simulink model "HD2_Driver_PY_v3"  (R2018a)
settings: Solver=ode1  StartTime=0.0  StopTime=inf  FixedStep=0.001  RelTol=1e-3  EnableMultiTasking=on
InitFcn:
  | % Assign block mask parameter to variable in base workspace
  | mdlPrefix_hd2_py = 'HD2_PY_';
  | mdlName_hd2_py = 'HD2_Driver_PY_v3';
  | blkName_hd2_py = 'HD2_Parameters';
  | blkRef_hd2_py = strcat(mdlName_hd2_py, '/', blkName_hd2_py);
  | 
  | % Extract list of parameters defined in the "HD2 Parameter" subsystem block
  | dialogParams_hd2_py = get_param( blkRef_hd2_py,'DialogParameters');
  | dialogParamsNames_hd2_py = fieldnames(dialogParams_hd2_py);
  | 
  | % Assign each parameter to a variable with mdlPrefix<param_name> formatted name
  | for idx = 1:numel(dialogParamsNames_hd2_py)
  |     paramVal = eval( get_param( blkRef_hd2_py, dialogParamsNames_hd2_py{idx} ) );
  |     assignin( 'base', strcat(mdlPrefix_hd2_py,dialogParamsNames_hd2_py{idx}), paramVal);
  | end
  | 
model workspace (MAT data in the model file):
  MCOS : class17 (value not decoded)
undefined symbols (not defined in the file): HD2_PY_CalibHome, HD2_PY_HandleLength, HD2_PY_HandleOffset, HD2_PY_HandleTol, HD2_PY_LinkLengths, HD2_PY_MotorAmpGains, HD2_PY_MotorAmpLimits, HD2_PY_QDirs, HD2_PY_QEnc, HD2_PY_QGains, HD2_PY_QKv, HIL, qc_get_step_size
libraries: quarc_library x30, simulink x10, simulink_extras x6
(part 2 of 2)

== matlab function HD2_Driver_PY_v3/Five Bar (PY) - Upper ==
  data: q input; Pos output; LinkLengths input; J output; R output
function [Pos, J, R] = FiveBarKinematics_PY(q, LinkLengths)
%#codegen

% This function computes the kinematics for a 5-Bar Mechanism (POSITIVE Y).

% The 5-Bar has three joints:
% Base Joint (q1): Defined to be rotating about the 5-Bar Native/Inertial x-axis
% First Joint (q2): Defined to be rotating about the local z-axis (when q1=0)
% Second Joint (q3): Also rotating about the local z-axis (when q1=0)
%
% The frames are defined such that when q=[0,0,0], the upper links are
% extending out towards the POSITIVE y direction (of the 5-Bar Native/Inertial frame) 
% while the base offset extends towards the positive x direction, forming a "L" shape.
%
% The LinkLengths contains 3 elements:
%
% L1 = Offset along x-axis of the q2 and q3 from origin
% L2 = Length of the link extending along local y-axis
% L3 = Length of final link from the joint to the end-effecter along local x-axis
%

s1 = sin(q(1));
c1 = cos(q(1));
s2 = sin(q(2));
c2 = cos(q(2));
s3 = sin(q(3));
c3 = cos(q(3));

L1 = LinkLengths(1);
L2 = LinkLengths(2);
L3 = LinkLengths(3);

% Position vector
x = L1 - L2*s2 - L3*s3;
y = L2*c1*c2 + L3*c1*c3;
z = L2*s1*c2 + L3*s1*c3;
Pos = [x, y, z]';

% Jacobian
J11 = 0;
J21 = -L2*s1*c2 - L3*s1*c3;
J31 = L2*c1*c2 + L3*c1*c3;

J12 = -L2*c2;
J22 = -L2*c1*s2;
J32 = -L2*s1*s2;

J13 = -L3*c3;
J23 = -L3*c1*s3;
J33 = -L3*s1*s3;

J = [ J11, J12, J13; J21, J22, J23; J31, J32, J33];

% Unit Base Vector of the end effector frame
% Rotation matrix from base frame (frame 0) to end effector frame (frame e)
% is defined as 
%
% r_0 = R . r_e
%
% where
%
% r_0 = vector expressed in base (5-Bar Native/Inertial) frame
% r_e = vector expressed in end effector frame
% R = [ unitX, unitY, unitZ ]
unitX = [ s3; -c1*c3; -s1*c3];
unitY = [ c3; c1*s3; s1*s3 ];
unitZ = [ 0; -s1; c1 ];
R = [unitX, unitY, unitZ];

== matlab function HD2_Driver_PY_v3/MATLAB Function ==
  data: unitZ input; R_upper input; qh output; R_lower input
function qh = HD2_Handle_Base_POSE(unitZ, R_upper, R_lower)
%#codegen

% Calculate the POSE of the handle base connector
% based on the direction unit vector between the two 5-bar EE.
% Assumption: the direction unit vector is in parallel with the handle axis
%
% qRoll_lower = Rotation angle along the final lower 5-bar link shaft (Roll)
% qPitch_lower = Rotation angle of the handle axis from the perpendicular position (Pitch)
% qRoll_upper = Rotation angle along the final upper 5-bar link shaft (Roll)
% qPitch_upper = Rotation angle of the handle axis from the perpendicular position (Pitch)
%


tol = eps;

% First, need to express the handle axis from HD^2 inertial frame to the
% 5-bar (lower) EE frame.
Zlower = R_lower' * unitZ;

if abs(Zlower(1)-1) < tol
    % Singular point, assign qRoll to 0 arbitrarily
    qRoll_lower = 0;
    qPitch_lower = sign(Zlower(1))*pi/2;
else
    qPitch_lower = asin(Zlower(1));
    if abs(Zlower(3)) < tol
        % Singular point, since qPitch == pi/2 is already covered before
        % qRoll must be either pi/2 or -pi/2
        qRoll_lower = -asin( Zlower(2)/cos(qPitch_lower) );
    else
        qRoll_lower = -atan2( Zlower(2), Zlower(3) );
    end
end

% Repeat for the upper 5-Bar
Zupper = R_upper' * unitZ;

if abs(Zupper(1)-1) < tol
    % Singular point, assign qRoll to 0 arbitrarily
    qRoll_upper = 0;
    qPitch_upper = sign(Zupper(1))*pi/2;
else
    qPitch_upper = asin(Zupper(1));
    if abs(Zupper(3)) < tol
        % Singular point, since qPitch == pi/2 is already covered before
        % qRoll must be either pi/2 or -pi/2
        qRoll_upper = -asin( Zupper(2)/cos(qPitch_upper) );
    else
        qRoll_upper = -atan2( Zupper(2), Zupper(3) );
    end
end


qh = [qRoll_lower qPitch_lower qRoll_upper qPitch_upper]';

== matlab function HD2_Driver_PY_v3/MATLAB Function1 ==
  data: qh input; qYaw input; x_lower input; xh output; R_hat input; Links input; L input; Rh output
function [xh, Rh]= HD2_End_Effecter_POSE(qh, qYaw, x_lower, R_hat, Links, L)
%#codegen

% Calculates the End Effecter POSE of the HD^2
% Based on the lower 5-Bar end effecter POSE
% and the handle base POSE
%
% L is the distance along the handle axis from
% the base of the handle to the handle End Effecter.
%
% Links contains the Link Lengths of the HD2
%
% Links(4) is the handle offset from the 5-Bar EE (default = 0.022m)

% Pre-calculate the trig functions
s1 = sin(qh(1));
c1 = cos(qh(1));
s2 = sin(qh(2));
c2 = cos(qh(2));
sY = sin(qYaw);
cY = cos(qYaw);

Loffset = Links(4);

% Unit Base Vector of the end effector frame
% Rotation matrix from base frame (frame 0) to end effector frame (frame e)
% is defined as 
%
% r_0 = R . r_e
%
% where
%
% r_0 = vector expressed in base (5-Bar Native/Inertial) frame
% r_e = vector expressed in end effector frame
% R = [ unitX, unitY, unitZ ]

% Basis vector w.r.t. to EE frame
xh_hat = [ c2, s1*s2, -c1*s2 ]';
yh_hat = [ 0, c1, s1 ]';
zh_hat = [ s2, -s1*c2, c1*c2 ]';


% Rotation matrix from 5-bar EE to handle EE
RhEE = [ xh_hat, yh_hat, zh_hat];

% Rotation matrix from HD^2 Native Frame to 5-bar EE Frame
% R_hat = [x_hat, y_hat, z_hat];

% Adding the yaw rotation to the handle EE frame to get the final EE frame.
RhEE_Yaw = [ cY, -sY, 0; sY, cY, 0; 0, 0, 1];

% Rotation matrix from HD^2 Native frame to handle EE
Rh = R_hat * RhEE *RhEE_Yaw;

% Position Vector w.r.t. 5-bar EE frame
x = L*s2 - Loffset*c2;
y = -L*s1*c2 - Loffset*s1*s2;
z = L*c1*c2 + Loffset*c1*s2;
xh = [x y z]';

% Position Vector w.r.t. HD^2 Native Frame
xh = x_lower + R_hat * xh;

== matlab function HD2_Driver_PY_v3/MATLAB Function2 ==
  data: W input; omega output; err output
function [omega, err]= ExtractAngularRateVector(W)
%#codegen

% Extract the angular rate vector from the skew symmetric matrix
%
% W = [   0, -wz,  wy ]
%     [  wz,   0, -wx ]
%     [ -wy,  wx,   0 ]

% Checking the diagonal entry to be zero.
% Flag the err signal if it is not.
if( norm(diag(W)) > 0.1 )
    err = 1;
else
    err = 0;
end

wx = W(3,2);
wy = W(1,3);
wz = W(2,1);
omega = [wx, wy, wz]';
